simulink model "Constant_Load_NoStim_mt2"  (Simulink 6.6)
settings: Solver=FixedStepDiscrete  StartTime=0.0  StopTime=inf  FixedStep=parameters.model.sample_time  RelTol=1e-3
values from neighbouring files (symbols this model uses):
  animation =     [FESCycling_30_PRE_CONST_loaded_12Aug2014_085817.mat]
  cad_ref = 30    [FESCycling_30_PRE_CONST_loaded_12Aug2014_085817.mat]    (also in constant_load_load.m = str2double(get(bla,'String')); constant_load_load_Orig.m = str2double(get(bla,'String')); param.m; param_orig.m = 0)
  freq_range = 1022.16    [FESCycling_30_PRE_CONST_loaded_12Aug2014_085817.mat]    (also in constant_load_load.m; constant_load_load_Orig.m = 466.8; param.m; param_orig.m = 865.41)
  freq_zero = -38.15    [FESCycling_30_PRE_CONST_loaded_12Aug2014_085817.mat]    (also in constant_load_load.m; constant_load_load_Orig.m = 116.7756; param.m; param_orig.m = 39.49)
  parameters =     [FESCycling_30_PRE_CONST_loaded_12Aug2014_085817.mat]
  phio_mat = [1 -0.559 0.0775]    [FESCycling_30_PRE_CONST_loaded_12Aug2014_085817.mat]    (also in constant_load_load.m; constant_load_load_Orig.m; param.m; param_orig.m)
  Pstep = 5    [FESCycling_30_PRE_CONST_loaded_12Aug2014_085817.mat]    (also in constant_load_load.m = str2double(get(bla,'String')); constant_load_load_Orig.m = str2double(get(bla,'String')); param.m = 32; param_orig.m = 114)
  Pw = 0    [FESCycling_30_PRE_CONST_loaded_12Aug2014_085817.mat]    (also in constant_load_load.m = str2double(get(bla,'String')); constant_load_load_Orig.m = str2double(get(bla,'String')); param.m; param_orig.m)
  ro_mat = [0.7602 -0.2976 0.0591]    [FESCycling_30_PRE_CONST_loaded_12Aug2014_085817.mat]    (also in constant_load_load.m; constant_load_load_Orig.m; param.m; param_orig.m)
  s_mat = [0.0005025 -0.0003467]    [FESCycling_30_PRE_CONST_loaded_12Aug2014_085817.mat]    (also in constant_load_load.m = [0.5025 -0.3467]*1e-3; constant_load_load_Orig.m = [0.5025 -0.3467]*1e-3; param.m = [0.5025 -0.3467]*1e-3; param_orig.m = [0.5025 -0.3467]*1e-3)
  slope = 15.81    [FESCycling_30_PRE_CONST_loaded_12Aug2014_085817.mat]    (also in constant_load_load.m; constant_load_load_Orig.m = 14.1374; param.m; param_orig.m = 14.1374)
  stim_max = 0.1    [FESCycling_30_PRE_CONST_loaded_12Aug2014_085817.mat]    (also in constant_load_load.m; constant_load_load_Orig.m; param.m = 500; param_orig.m = 0)
  stim_min = 0    [FESCycling_30_PRE_CONST_loaded_12Aug2014_085817.mat]    (also in constant_load_load.m; constant_load_load_Orig.m; param.m; param_orig.m)
  t_mat = [0.0002987 -0.000166 2.31e-05]    [FESCycling_30_PRE_CONST_loaded_12Aug2014_085817.mat]    (also in constant_load_load.m = [0.2987 -0.1660 0.0231]*1e-3; constant_load_load_Orig.m = [0.2987 -0.1660 0.0231]*1e-3; param.m = [0.2987 -0.1660 0.0231]*1e-3; param_orig.m = [0.2987 -0.1660 0.0231]*1e-3)
  Ts = 20    [FESCycling_30_PRE_CONST_loaded_12Aug2014_085817.mat]    (also in constant_load_load.m; constant_load_load_Orig.m; param.m; param_orig.m)
  Tw = 6000    [FESCycling_30_PRE_CONST_loaded_12Aug2014_085817.mat]    (also in constant_load_load.m; constant_load_load_Orig.m; param.m; param_orig.m)
undefined symbols (not defined in the file or in its folder): ansim
libraries: ni_lib x2, Stimulation_Currents_lib x1, stimulation_staticAngles_lib x1
settings Model: Tag=D:\Ben\Matlab_Files\my_FES_Stuff\FES_Cycling_Models\Parameter_Files\GLA_BEN_Params_3.m  Creator=research  LastModifiedBy=research
settings DataIOCC: SignalLoggingName=sigsOut
settings OptimizationCC: BooleanDataType=off
settings DebuggingCC: SignalResolutionControl=TryResolveAllWithWarning  SolverPrmCheckMsg=none  MultiTaskDSMMsg=warning  MultiTaskCondExecSysMsg=none  StrictBusMsg=None
settings HardwareCC: TargetUnknown=on
settings RTWCC: IncludeERTFirstTime=on

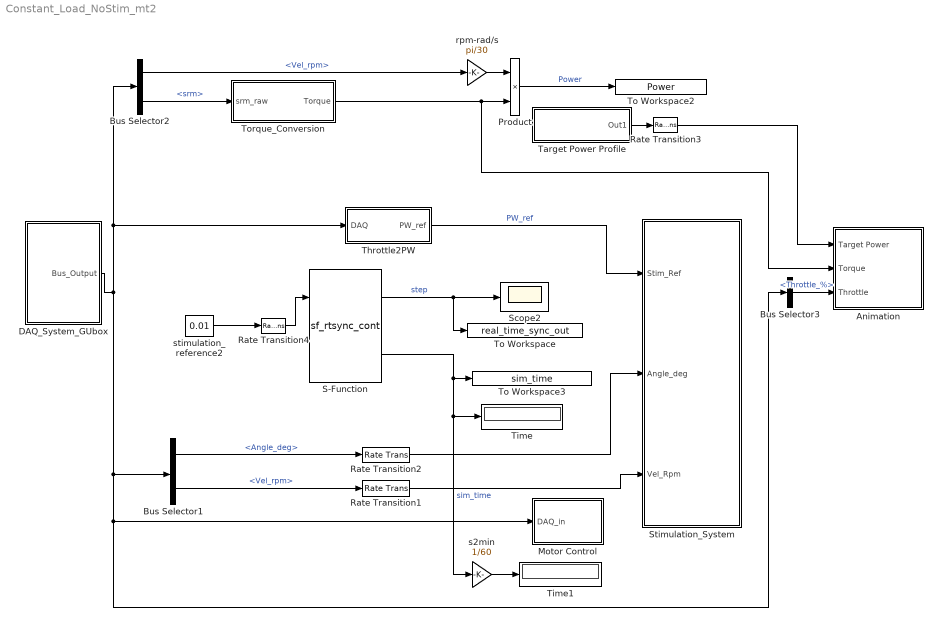
== system Constant_Load_NoStim_mt2 ==
  Animation : Subsystem
  Bus Selector1 : BusSelector  OutputSignals=Angle_deg,Vel_rpm
  Bus Selector2 : BusSelector  OutputSignals=Vel_rpm,srm
  Bus Selector3 : BusSelector  OutputSignals=Throttle_%
  DAQ_System_GUbox : Subsystem
  Motor Control : Subsystem
  Product : Product  SaturateOnIntegerOverflow=on
  Rate Transition1 : RateTransition  OutPortSampleTime=parameters.model.sample_time
  Rate Transition2 : RateTransition  OutPortSampleTime=parameters.model.sample_time
  Rate Transition3 : RateTransition  OutPortSampleTime=parameters.sample_time
  Rate Transition4 : RateTransition  X0=0.011  OutPortSampleTime=parameters.model.sample_time
  S-Function : S-Function  FunctionName=sf_rtsync_cont  Parameters=1
  Scope2 : Scope
      settings: YMin=-3.46945e-018  YMax=0.12
  Stimulation_System : Subsystem
  Target Power Profile : Subsystem
  Throttle2PW : Subsystem
  Time : Display
  Time1 : Display
  To Workspace : ToWorkspace  VariableName=real_time_sync_out  SampleTime=parameters.model.sample_time  SaveFormat=Array
  To Workspace2 : ToWorkspace  VariableName=Power  SampleTime=parameters.sample_time  SaveFormat=Array
  To Workspace3 : ToWorkspace  VariableName=sim_time  SampleTime=-1  SaveFormat=Array
      settings: Decimation=5
  Torque_Conversion : Subsystem
  rpm-rad/s : Gain  Gain=pi/30  SaturateOnIntegerOverflow=on
  s2min : Gain  Gain=1/60  SaturateOnIntegerOverflow=on
  stimulation_reference2 : Constant  Value=0.01
      mask Type: text(0.5,0.5,'bla_name.bla', 'VerticalAlignment', 'middle', 'HorizontalAlignment', 'centre')
  wires:
  Bus Selector1/2 -> Rate Transition1/1  "<Vel_rpm>"
  Bus Selector1/1 -> Rate Transition2/1  "<Angle_deg>"
  Bus Selector2/2 -> Torque_Conversion/1(srm_raw)  "<srm>"
  DAQ_System_GUbox/1(Bus_Output) -> Bus Selector1/1, Motor Control/1(DAQ_in), Bus Selector3/1, Bus Selector2/1, Throttle2PW/1(DAQ)
  Rate Transition1/1 -> Stimulation_System/3(Vel_Rpm)
  Rate Transition2/1 -> Stimulation_System/2(Angle_deg)
  S-Function/2 -> To Workspace3/1, Time/1, s2min/1  "sim_time"
  S-Function/1 -> Scope2/1, To Workspace/1  "step"
  Rate Transition4/1 -> S-Function/1
  stimulation_reference2/1 -> Rate Transition4/1
  s2min/1 -> Time1/1
  Torque_Conversion/1(Torque) -> Product/2, Animation/2(Torque)
  rpm-rad/s/1 -> Product/1
  Bus Selector2/1 -> rpm-rad/s/1  "<Vel_rpm>"
  Target Power Profile/1(Out1) -> Rate Transition3/1
  Product/1 -> To Workspace2/1  "Power"
  Rate Transition3/1 -> Animation/1(Target Power)
  Bus Selector3/1 -> Animation/3(Throttle)  "<Throttle_%>"
  Throttle2PW/1(PW_ref) -> Stimulation_System/1(Stim_Ref)  "PW_ref"

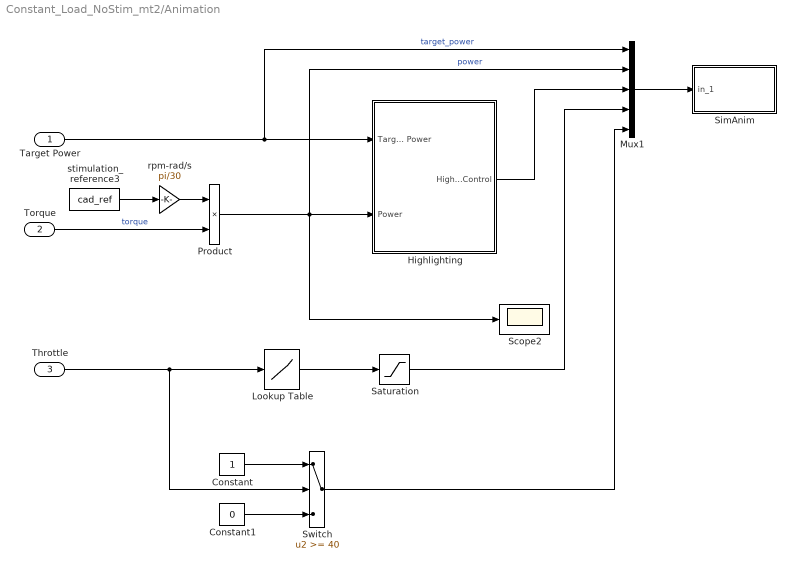
== system Constant_Load_NoStim_mt2/Animation ==
  Target Power : Inport
  Torque : Inport  Port=2
  Throttle : Inport  Port=3
  Constant : Constant
  Constant1 : Constant  Value=0
  Highlighting : Subsystem
  Lookup Table : Lookup  InputValues=[0 40 100]  OutputValues=[-5 0 19.9]
  Mux1 : Mux  Inputs=5
  Product : Product  SaturateOnIntegerOverflow=on
  Saturation : Saturate  UpperLimit=19.9  LowerLimit=-5
  Scope2 : Scope
      settings: TimeRange=2000  YMin=-2  YMax=60  SaveName=ScopeData6
  SimAnim : Subsystem
      settings: NameChangeFcn=ansim([],[],[],'NameChange');  OpenFcn=ansimini #Initialize
      mask Type: Simulation Animation
      mask Help: cal2.mat
      mask Display: disp('Simulation\nAnimation')
  Switch : Switch  Threshold=40
  rpm-rad/s : Gain  Gain=pi/30  SaturateOnIntegerOverflow=on
  stimulation_reference3 : Constant  Value=cad_ref
      mask Type: text(0.5,0.5,'bla_name.bla', 'VerticalAlignment', 'middle', 'HorizontalAlignment', 'centre')
  wires:
  Mux1/1 -> SimAnim/1(in_1)
  Target Power/1 -> Highlighting/1(Target Power), Mux1/1  "target_power"
  Highlighting/1(Highlight Control) -> Mux1/3
  Lookup Table/1 -> Saturation/1
  Saturation/1 -> Mux1/4
  Throttle/1 -> Lookup Table/1, Switch/2
  Constant/1 -> Switch/1
  Constant1/1 -> Switch/3
  Switch/1 -> Mux1/5
  rpm-rad/s/1 -> Product/1
  Product/1 -> Mux1/2, Highlighting/2(Power), Scope2/1  "power"
  Torque/1 -> Product/2  "torque"
  stimulation_reference3/1 -> rpm-rad/s/1

== system Constant_Load_NoStim_mt2/DAQ_System_GUbox ==
  note: Angle velocity (cadence) is more
      | useful in rpm (revolutions per
      | minute) so devide deg/s by 6.
  note: Convert the angle from between
      | 0 and 1 to between 0 and 360
      | and calculate the rate of change
      | of the angle in deg/s.
  Angle Conversion : Subsystem
  Bus Creator : BusCreator
  Bus Selector1 : BusSelector  OutputSignals=shaft_encoder_raw
  Bus Selector3 : BusSelector  OutputSignals=throttle_raw
  Gain1 : Gain  Gain=1/6  SaturateOnIntegerOverflow=on
  Hardware Interface via GU box : Subsystem
  Output Signal Conversion : Subsystem
  Output Signal Conversion2 : Subsystem
  Throttle Valuation : Subsystem
  To Workspace1 : ToWorkspace  VariableName=angle_deg  SampleTime=-1  SaveFormat=Array
  To Workspace2 : ToWorkspace  VariableName=vel_rpm  SampleTime=-1  SaveFormat=Array
  Bus_Output : Outport
  wires:
  Output Signal Conversion2/1(Out = 0 to 1) -> Throttle Valuation/1(throttle (0 to 1))
  Gain1/1 -> To Workspace2/1, Bus Creator/2  "Vel_rpm"
  Angle Conversion/2(Vel (deg/s)) -> Gain1/1
  Output Signal Conversion/1(Out = 0 to 1) -> Angle Conversion/1(Angle (0 to 1 volts))
  Bus Selector1/1 -> Output Signal Conversion/1(In = 0 to 5)  "<shaft_encoder_raw>"
  Bus Selector3/1 -> Output Signal Conversion2/1(In = 0 to 5)  "<throttle_raw>"
  Angle Conversion/1(Angle (deg)) -> To Workspace1/1, Bus Creator/1  "Angle_deg"
  Throttle Valuation/1(Throttle_%) -> Bus Creator/3  "Throttle_%"
  Hardware Interface via GU box/1(Hardware_Out_1) -> Bus Selector1/1, Bus Selector3/1
  Hardware Interface via GU box/2(Hardware_Out_3) -> Bus Creator/4  "srm"
  Bus Creator/1 -> Bus_Output/1

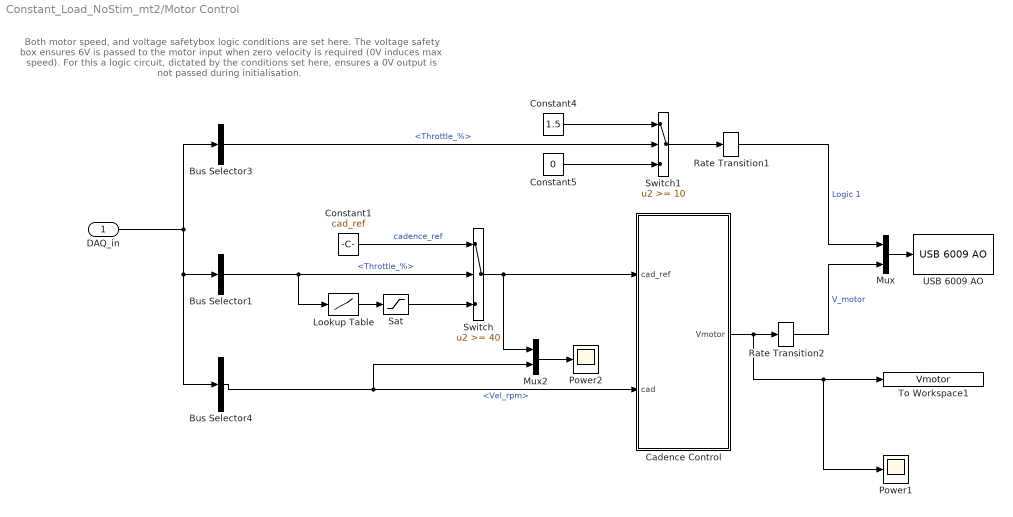
== system Constant_Load_NoStim_mt2/Motor Control ==
  note: Both motor speed, and voltage safetybox logic conditions are set here.
      | The voltage safety box ensures 6V is passed to the motor input when
      | zero velocity is required (0V induces max speed). For this a logic circuit,
      | dictated by the conditions set here, ensures a 0V output is not passed
      | during initialisation.
  DAQ_in : Inport
  Bus Selector1 : BusSelector  OutputSignals=Throttle_%
  Bus Selector3 : BusSelector  OutputSignals=Throttle_%
  Bus Selector4 : BusSelector  OutputSignals=Vel_rpm
  Cadence Control : Subsystem
  Constant1 : Constant  Value=cad_ref  SampleTime=-1
  Constant4 : Constant  Value=1.5
  Constant5 : Constant  Value=0
  Lookup Table : Lookup  InputValues=[10 40]  OutputValues=[0 cad_ref]  LookUpMeth=Interpolation-Use End Values
  Mux : Mux  Inputs=2
  Mux2 : Mux  Inputs=2
  Power1 : Scope
      settings: TimeRange=1000  YMin=0  SaveName=ScopeData3
  Power2 : Scope
      settings: TimeRange=1000  YMin=0  YMax=100  SaveName=ScopeData5
  Rate Transition1 : RateTransition  OutPortSampleTime=20
  Rate Transition2 : RateTransition  OutPortSampleTime=20
  Sat : Saturate  UpperLimit=cad_ref  LowerLimit=0
  Switch : Switch  Threshold=40
  Switch1 : Switch  Threshold=10
  To Workspace1 : ToWorkspace  VariableName=Vmotor  SampleTime=parameters.sample_time  SaveFormat=Array
  USB 6009 AO : ni_lib/USB 6009 AO  channels=[2 1]  Ts=20  inp_min=0  inp_max=5
  wires:
  DAQ_in/1 -> Bus Selector3/1, Bus Selector4/1, Bus Selector1/1
  Mux2/1 -> Power2/1
  Mux/1 -> USB 6009 AO/1
  Constant5/1 -> Switch1/3
  Switch1/1 -> Rate Transition1/1
  Constant4/1 -> Switch1/1
  Rate Transition1/1 -> Mux/1  "Logic 1"
  Rate Transition2/1 -> Mux/2  "V_motor"
  Bus Selector3/1 -> Switch1/2  "<Throttle_%>"
  Bus Selector4/1 -> Cadence Control/2(cad), Mux2/2  "<Vel_rpm>"
  Cadence Control/1(Vmotor) -> Rate Transition2/1, To Workspace1/1, Power1/1
  Switch/1 -> Cadence Control/1(cad_ref), Mux2/1
  Constant1/1 -> Switch/1  "cadence_ref"
  Bus Selector1/1 -> Switch/2, Lookup Table/1  "<Throttle_%>"
  Lookup Table/1 -> Sat/1
  Sat/1 -> Switch/3

== system Constant_Load_NoStim_mt2/Stimulation_System ==
  Stim_Ref : Inport
  Angle_deg : Inport  Port=2
  Vel_Rpm : Inport  Port=3
  Serial_Stimulation_System : Subsystem
  wires:
  Stim_Ref/1 -> Serial_Stimulation_System/1(Stim_ref)
  Angle_deg/1 -> Serial_Stimulation_System/2(Angle_deg)
  Vel_Rpm/1 -> Serial_Stimulation_System/3(Vel_rpm)

== system Constant_Load_NoStim_mt2/Target Power Profile ==
  Step : Step  Time=Tw  Before=Pw  After=Pw + Pstep  SampleTime=0
  Out1 : Outport
  wires:
  Step/1 -> Out1/1

== system Constant_Load_NoStim_mt2/Throttle2PW ==
  DAQ : Inport
  Bus Selector3 : BusSelector  OutputSignals=Throttle_%
  Lookup Table2 : Lookup  InputValues=[0 20 40 100]  OutputValues=[0 0 stim_min stim_max]  LookUpMeth=Interpolation-Use End Values
  Mux1 : Mux  Inputs=2
  Rate Transition1 : RateTransition  OutPortSampleTime=parameters.model.sample_time
  Saturation : Saturate  UpperLimit=stim_max  LowerLimit=0
  PW_ref : Outport
  wires:
  DAQ/1 -> Bus Selector3/1
  Bus Selector3/1 -> Rate Transition1/1  "<Throttle_%>"
  Mux1/1 -> PW_ref/1
  Rate Transition1/1 -> Lookup Table2/1
  Lookup Table2/1 -> Saturation/1
  Saturation/1 -> Mux1/1, Mux1/2  "pw_h_g"

== system Constant_Load_NoStim_mt2/Torque_Conversion ==
  srm_raw : Inport
  Discrete Transfer Fcn : DiscreteTransferFcn  Numerator="[0.0051    0.0101    0.0051]"  Denominator="[1.0000   -1.7889    0.8092]"  SampleTime=parameters.sample_time
  Mux : Mux  Inputs=2
  Normalise srm raw : Gain  Gain=1/5  SaturateOnIntegerOverflow=on
  SRM frequency - Voltage1 : Subsystem
  To Workspace2 : ToWorkspace  VariableName=Torque  SampleTime=parameters.sample_time  SaveFormat=Array
  torque : Scope
      settings: YMin=8.95  YMax=9.6  SaveName=ScopeData4
  Torque : Outport
  wires:
  srm_raw/1 -> Normalise srm raw/1
  SRM frequency - Voltage1/1(Torque (Nm)) -> Mux/1, Discrete Transfer Fcn/1  "torque_raw"
  Mux/1 -> torque/1
  Discrete Transfer Fcn/1 -> Mux/2, To Workspace2/1, Torque/1  "torque_(filtered)"
  Normalise srm raw/1 -> SRM frequency - Voltage1/1(In 0 to 1)

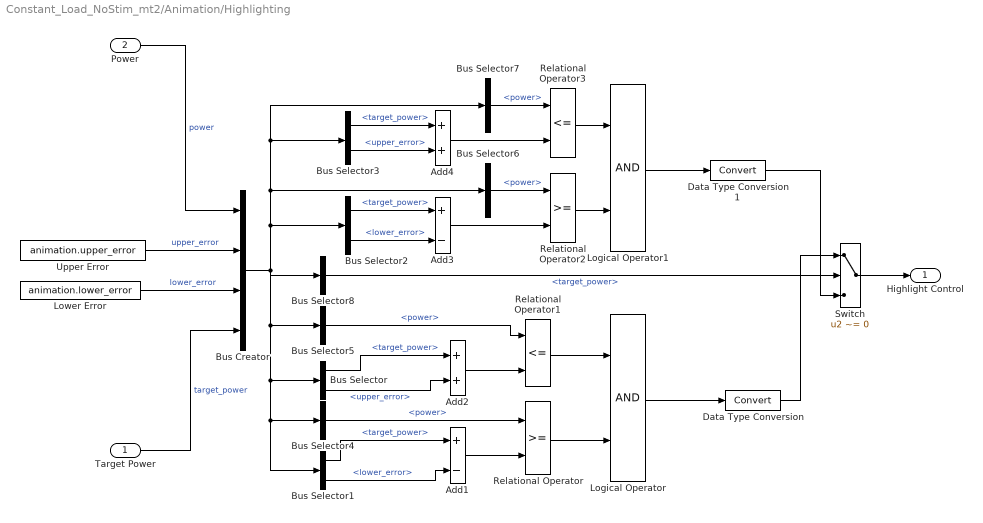
== system Constant_Load_NoStim_mt2/Animation/Highlighting ==
  Target Power : Inport
  Power : Inport  Port=2
  Add1 : Sum  Inputs=+-  OutScaling=2^-10
  Add2 : Sum  OutScaling=2^-10
  Add3 : Sum  Inputs=+-  OutScaling=2^-10
  Add4 : Sum  OutScaling=2^-10
  Bus Creator : BusCreator
  Bus Selector : BusSelector  OutputSignals=target_power,upper_error
  Bus Selector1 : BusSelector  OutputSignals=target_power,lower_error
  Bus Selector2 : BusSelector  OutputSignals=target_power,lower_error
  Bus Selector3 : BusSelector  OutputSignals=target_power,upper_error
  Bus Selector{4..7} (4 alike) : BusSelector  OutputSignals=power
  Bus Selector8 : BusSelector  OutputSignals=target_power
  Data Type Conversion : DataTypeConversion  OutDataTypeMode=double
  Data Type Conversion1 : DataTypeConversion  OutDataTypeMode=double
  Logical Operator : Logic  AllPortsSameDT=off  OutDataTypeMode=Boolean
  Logical Operator1 : Logic  AllPortsSameDT=off  OutDataTypeMode=Boolean
  Lower Error : Constant  Value=animation.lower_error
  Relational Operator : RelationalOperator  LogicOutDataTypeMode=Boolean
  Relational Operator1 : RelationalOperator  Operator=<=  LogicOutDataTypeMode=Boolean
  Relational Operator2 : RelationalOperator  LogicOutDataTypeMode=Boolean
  Relational Operator3 : RelationalOperator  Operator=<=  LogicOutDataTypeMode=Boolean
  Switch : Switch  Criteria=u2 ~= 0
  Upper Error : Constant  Value=animation.upper_error
  Highlight Control : Outport
  wires:
  Relational Operator/1 -> Logical Operator/2
  Logical Operator/1 -> Data Type Conversion/1
  Data Type Conversion/1 -> Switch/1
  Add1/1 -> Relational Operator/2
  Relational Operator3/1 -> Logical Operator1/1
  Relational Operator2/1 -> Logical Operator1/2
  Add4/1 -> Relational Operator3/2
  Add3/1 -> Relational Operator2/2
  Target Power/1 -> Bus Creator/4  "target_power"
  Bus Selector/1 -> Add2/1  "<target_power>"
  Bus Selector/2 -> Add2/2  "<upper_error>"
  Bus Creator/1 -> Bus Selector2/1, Bus Selector6/1, Bus Selector3/1, Bus Selector7/1, Bus Selector/1, Bus Selector4/1, Bus Selector1/1, Bus Selector5/1, Bus Selector8/1
  Bus Selector1/1 -> Add1/1  "<target_power>"
  Bus Selector1/2 -> Add1/2  "<lower_error>"
  Bus Selector2/1 -> Add3/1  "<target_power>"
  Bus Selector2/2 -> Add3/2  "<lower_error>"
  Bus Selector3/1 -> Add4/1  "<target_power>"
  Bus Selector3/2 -> Add4/2  "<upper_error>"
  Lower Error/1 -> Bus Creator/3  "lower_error"
  Upper Error/1 -> Bus Creator/2  "upper_error"
  Bus Selector7/1 -> Relational Operator3/1  "<power>"
  Bus Selector6/1 -> Relational Operator2/1  "<power>"
  Bus Selector5/1 -> Relational Operator1/1  "<power>"
  Bus Selector4/1 -> Relational Operator/1  "<power>"
  Logical Operator1/1 -> Data Type Conversion1/1
  Bus Selector8/1 -> Switch/2  "<target_power>"
  Data Type Conversion1/1 -> Switch/3
  Switch/1 -> Highlight Control/1
  Add2/1 -> Relational Operator1/2
  Relational Operator1/1 -> Logical Operator/1
  Power/1 -> Bus Creator/1  "power"

== system Constant_Load_NoStim_mt2/Animation/SimAnim ==
  in_1 : Inport
  Terminator : Terminator
  ansim : S-Function  LoadFcn=ansim([],[],[],'LoadBlock');  StartFcn=ansim([],[],[],'Start');  StopFcn=ansim([],[],[],'Stop');  FunctionName=ansim  Parameters=1
      settings: CopyFcn=ansim([],[],[],'CopyBlock');  DeleteFcn=ansim([],[],[],'DeleteBlock');
  wires:
  in_1/1 -> ansim/1
  ansim/1 -> Terminator/1

== system Constant_Load_NoStim_mt2/DAQ_System_GUbox/Angle Conversion ==
  note: This system converts an
      | angle described as a voltage
      | between 0 and 1 and turns it
      | into an angle in degrees.
      | The rate of change of angle
      | is also calculated.
  note: Ensure that the final angle
      | value is between 0 and 360
  note: Use this constant input
      | when the 0 point of the
      | input angle is not the same
      | as the 0 point needed by
      | the rest of the simulaink
      | model.
      | (left leg horizontally forward)
  note: Angle Conversion
  Angle (0 to 1 volts) : Inport
  0 < u < 360 : Fcn  Expr=u - 360*floor(u/360)
  Angle Derivative : Subsystem  mask(AngleDer){Tdf=0.5, Ts=5}
      mask prompts: Tdf "Filter constant"; Ts "Sampling Time"
      mask help:
      | This block calculates the angular velocity from the angle measuremet.  If the input angle is in degrees then the output velocity is in deg/s.  The block takes account of the transition from 359 deg to 0 deg or vice versa and computes the derivative based on the sample time given  The output is passed through a low pass filter based on the fliter constant also given.
      |
      | Implemented by Nils-Otto Negaard
      | Documented by Ben Saunders (17/06/2003)
  Angle Shift : Constant  Value=parameters.angle_shift
  Sum : Sum  Inputs=++|  SaturateOnIntegerOverflow=on  InputSameDT=on
  angle into degrees : Fcn  Expr=u*360
  Angle (deg) : Outport
  Vel (deg/s) : Outport  Port=2
  wires:
  angle into degrees/1 -> Angle Derivative/1(Angle), Sum/2
  Sum/1 -> 0 < u < 360/1
  0 < u < 360/1 -> Angle (deg)/1
  Angle (0 to 1 volts)/1 -> angle into degrees/1
  Angle Derivative/1(Vel (deg/s)) -> Vel (deg/s)/1
  Angle Shift/1 -> Sum/1

== system Constant_Load_NoStim_mt2/DAQ_System_GUbox/Hardware Interface via GU box ==
  note: Hardware Interface (via USB-6009)
  Bus Creator : BusCreator
  Demux1 : Demux  Outputs=5
  To Workspace1 : ToWorkspace  VariableName=throttle_raw  SampleTime=-1  SaveFormat=Array
  To Workspace2 : ToWorkspace  VariableName=srm_cad  SampleTime=-1  SaveFormat=Array
  To Workspace3 : ToWorkspace  VariableName=torque_dig  SampleTime=-1  SaveFormat=Array
  To Workspace4 : ToWorkspace  VariableName=torque_ana  SampleTime=-1  SaveFormat=Array
  To Workspace5 : ToWorkspace  VariableName=shaft_encoder_raw  SampleTime=-1  SaveFormat=Array
  USB 6009 AI : ni_lib/USB 6009 AI  channels=[1 2 3 4 5]  Ts=5  inp_min=-5  inp_max=5  terminalcfg=RSE
  Hardware_Out_1 : Outport
  Hardware_Out_3 : Outport  Port=2
  wires:
  Bus Creator/1 -> Hardware_Out_1/1
  Demux1/2 -> Bus Creator/2, To Workspace1/1  "throttle_raw"
  Demux1/5 -> To Workspace2/1  "srm_cadence"
  USB 6009 AI/1 -> Demux1/1
  Demux1/4 -> Bus Creator/4, To Workspace3/1  "torque_dig"
  Demux1/3 -> To Workspace4/1, Hardware_Out_3/1, Bus Creator/3  "torque_ana"
  Demux1/1 -> Bus Creator/1, To Workspace5/1  "shaft_encoder_raw"

== system Constant_Load_NoStim_mt2/DAQ_System_GUbox/Output Signal Conversion ==
  In = 0 to 5 : Inport
  Constant : Constant  Value=0
  Gain4 : Gain  Gain=1/5  SaturateOnIntegerOverflow=on
  Sum : Sum  Inputs=++|  SaturateOnIntegerOverflow=on  InputSameDT=on
  Out = 0 to 1 : Outport
  wires:
  In = 0 to 5/1 -> Gain4/1
  Sum/1 -> Out = 0 to 1/1
  Constant/1 -> Sum/1
  Gain4/1 -> Sum/2

== system Constant_Load_NoStim_mt2/DAQ_System_GUbox/Output Signal Conversion2 ==
  In = 0 to 5 : Inport
  Constant : Constant  Value=0
  Gain4 : Gain  Gain=1/5  SaturateOnIntegerOverflow=on
  Sum : Sum  Inputs=++|  SaturateOnIntegerOverflow=on  InputSameDT=on
  Out = 0 to 1 : Outport
  wires:
  In = 0 to 5/1 -> Gain4/1
  Sum/1 -> Out = 0 to 1/1
  Constant/1 -> Sum/1
  Gain4/1 -> Sum/2

== system Constant_Load_NoStim_mt2/DAQ_System_GUbox/Throttle Valuation ==
  note: Throttle Valuation
  note: This Subsystem is used to
      | scale the throttle signal from
      | an input of 0 to 1 to a
      | percentage (0 to 100).  Since
      | the throttle does not always
      | show 0 when let go, it is
      | forced to 0 using the validity
      | signal. This is a safty
      | consideration.  Note that
      | when the throttle switch is on
      | then the validity signal still
      | goes to 0 when the throttle
      | has been let go.
  throttle (0 to 1) : Inport
  Gain3 : Gain  Gain=100  SaturateOnIntegerOverflow=on
  Throttle_% : Outport
  wires:
  Gain3/1 -> Throttle_%/1  "Throttle_%"
  throttle (0 to 1)/1 -> Gain3/1

== system Constant_Load_NoStim_mt2/Motor Control/Cadence Control ==
  cad_ref : Inport
  cad : Inport  Port=2
  Gain1 : Gain  Gain=6  SaturateOnIntegerOverflow=on
  Gain2 : Gain  Gain=6  SaturateOnIntegerOverflow=on
  Lookup Table : Lookup  InputValues=[0 1]  OutputValues=[2.5 1.25]
  Rate Transition1 : RateTransition  OutPortSampleTime=parameters.sample_time
  rstcon antireset2 : Subsystem
  Vmotor : Outport
  wires:
  rstcon antireset2/1(Vm_ref) -> Lookup Table/1
  cad/1 -> Gain1/1
  Gain2/1 -> rstcon antireset2/1(cad_ref)
  cad_ref/1 -> Gain2/1
  Lookup Table/1 -> Rate Transition1/1
  Gain1/1 -> rstcon antireset2/2(cad_act)
  Rate Transition1/1 -> Vmotor/1

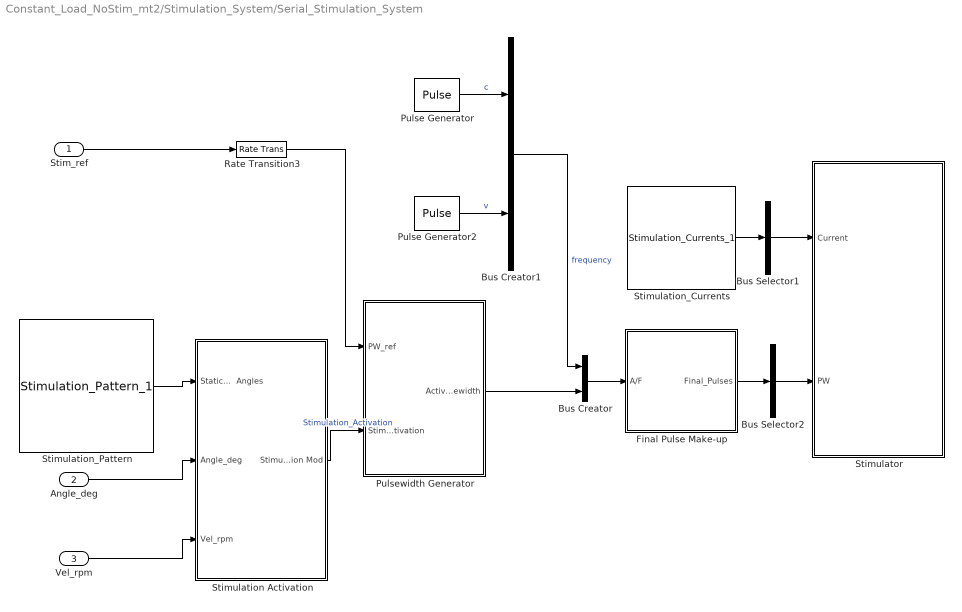
== system Constant_Load_NoStim_mt2/Stimulation_System/Serial_Stimulation_System ==
  Stim_ref : Inport
  Angle_deg : Inport  Port=2
  Vel_rpm : Inport  Port=3
  Bus Creator : BusCreator  Inputs=2
  Bus Creator1 : BusCreator  Inputs=2
  Bus Selector1 : BusSelector  OutputSignals=R.Quad,R.Ham,R.Glut,L.Quad,L.Ham,L.Glut  OutputAsBus=on
  Bus Selector2 : BusSelector  OutputSignals=R.Quad_r,R.Ham_r,R.Glut_r,L.Quad_l,L.Ham_l,L.Glut_l  OutputAsBus=on
  Final Pulse Make-up : Subsystem
  Pulse Generator : DiscretePulseGenerator  Period=3
  Pulse Generator2 : DiscretePulseGenerator  Period=3
  Pulsewidth Generator : Subsystem
  Rate Transition3 : RateTransition  OutPortSampleTime=parameters.model.sample_time
  Stimulation Activation : Subsystem
  Stimulation_Currents : Stimulation_Currents_lib/Stimulation_Currents_1  SystemSampleTime=-1  Quad_R=40  Ham_R=0  Glut_R=0  Calf_R=0  ExactOpp=on  Quad_L=[40]  Ham_L=[0]  Glut_L=[0]  Calf_L=[0]
  Stimulation_Pattern : stimulation_staticAngles_lib/Stimulation_Pattern_1  SystemSampleTime=-1  Quad_R=[55 155]  Ham_R=[188 265]  Glut_R=[90 180]  Calf_R=[180 205]  ExactOpp=on  Quad_L="[235  335]"  Ham_L="[8  85]"  Glut_L="[270    0]"  Calf_L="[0  25]"
  Stimulator : Subsystem
  wires:
  Stimulation Activation/1(Stimulation  Activation Mod) -> Pulsewidth Generator/2(Stimulation Activation)  "Stimulation_Activation"
  Stimulation_Pattern/1 -> Stimulation Activation/1(Static  Stimulation  Angles)
  Angle_deg/1 -> Stimulation Activation/2(Angle_deg)
  Vel_rpm/1 -> Stimulation Activation/3(Vel_rpm)
  Stimulation_Currents/1 -> Bus Selector1/1
  Stim_ref/1 -> Rate Transition3/1
  Rate Transition3/1 -> Pulsewidth Generator/1(PW_ref)
  Bus Selector1/1 -> Stimulator/1(Current)
  Bus Selector2/1 -> Stimulator/2(PW)
  Pulse Generator2/1 -> Bus Creator1/2  "v"
  Pulse Generator/1 -> Bus Creator1/1  "c"
  Bus Creator1/1 -> Bus Creator/1  "frequency"
  Final Pulse Make-up/1(Final_Pulses) -> Bus Selector2/1
  Bus Creator/1 -> Final Pulse Make-up/1(A/F)
  Pulsewidth Generator/1(Activation/Pulsewidth) -> Bus Creator/2

== system Constant_Load_NoStim_mt2/Torque_Conversion/SRM frequency - Voltage1 ==
  note: Convert frequency to Torque (Nm)
      |
      | The data for this can be gained
      | from the SRM sensot itself. The
      | ZOPM (Zero Offset of the Power
      | Meter) is calculated and displayed
      | by the SRM meter.  Please check
      | the SRM manual for details. The
      | 'Slope' value can be read from the
      | back of the SRM sensor.
  note: SRM Frequency to Voltage
  note: This system reads in a 0 to 1 voltage
      | from an AD card that comes from a
      | frequency to voltage converter.  The
      | frequency signal comes from the SRM
      | sensor meter.  In order to work out the
      | torque on the sensor the process has
      | to be reversed.  Thus the voltage has
      | to be converted back into a frequency
      | and then back into a torque.
  note: Convert signal to frequency
      |
      | The frequency to voltage converter
      | was designed (at Glasgow by
      | Gordon) such that 0 volts = 300 Hz
      | and 5 volts = 1000 Hz.  The
      | mapping is linear.
  note: The final signal is filtered.
      | This may have a relatively
      | large rise time so that
      | cyclinc pedal forces are
      | smoothrd out. (ie forces at
      | 90 deg will always be
      | different to forces at 180
      | deg).
  In 0 to 1 : Inport
  1 / Slope1 : Constant  Value=1/slope
  Frequency Range : Constant  Value=freq_range
  Product : Product  SaturateOnIntegerOverflow=on  InputSameDT=on
  Product1 : Product  SaturateOnIntegerOverflow=on  InputSameDT=on
  Sum : Sum  Inputs=|++  SaturateOnIntegerOverflow=on  InputSameDT=on
  Sum1 : Sum  Inputs=-+|  SaturateOnIntegerOverflow=on  InputSameDT=on
  Sum2 : Sum  Inputs=-+|  SaturateOnIntegerOverflow=on  InputSameDT=on
  ZOPM : Constant  Value=parameters.srm_conversion.ZOPM
  Zero Frequency : Constant  Value=freq_zero
  offset : Constant  Value=-9
  Torque (Nm) : Outport
  wires:
  Zero Frequency/1 -> Sum/2
  1 / Slope1/1 -> Product1/2
  ZOPM/1 -> Sum2/1
  Frequency Range/1 -> Product/1
  Sum/1 -> Sum2/2  "frequency"
  In 0 to 1/1 -> Product/2
  Product/1 -> Sum/1
  Sum2/1 -> Product1/1
  Product1/1 -> Sum1/2  "Nm"
  Sum1/1 -> Torque (Nm)/1
  offset/1 -> Sum1/1

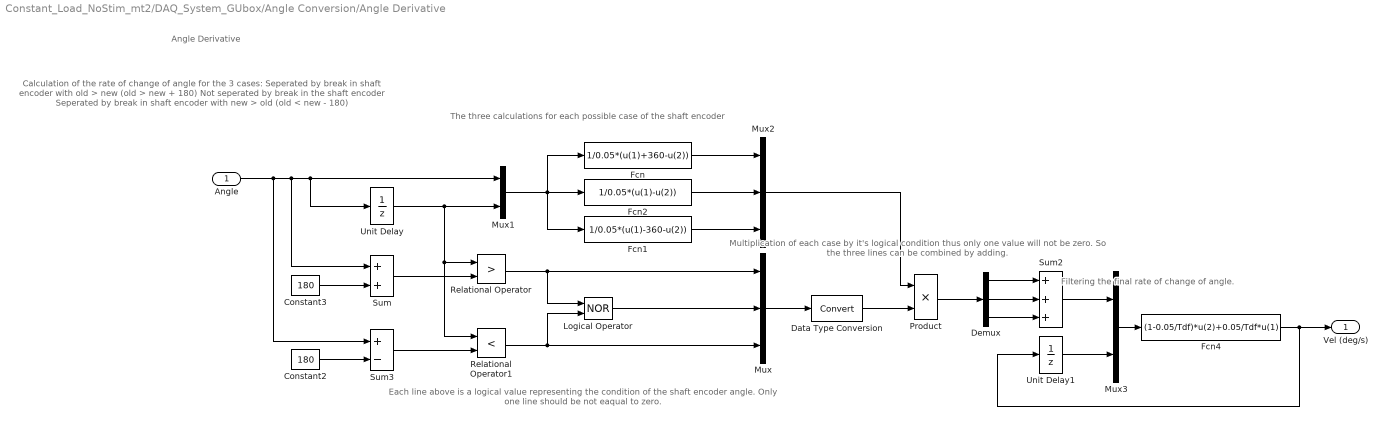
== system Constant_Load_NoStim_mt2/DAQ_System_GUbox/Angle Conversion/Angle Derivative ==
  note: Calculation of the rate of change of angle
      | for the 3 cases:
      | Seperated by break in shaft encoder with old > new (old > new + 180)
      | Not seperated by break in the shaft encoder
      | Seperated by break in shaft encoder with new > old (old < new - 180)
  note: Each line above is a logical value
      | representing the condition of the
      | shaft encoder angle.  Only one line
      | should be not eaqual to zero.
  note: The three calculations for each
      | possible case of the shaft encoder
  note: Multiplication of each case
      | by it's logical condition thus
      | only one value will not be zero.
      | So the three lines can be
      | combined by adding.
  note: Filtering the final rate of
      | change of angle.
  note: Angle Derivative
  Angle : Inport
  Constant2 : Constant  Value=180  VectorParams1D=off
  Constant3 : Constant  Value=180  VectorParams1D=off
  Data Type Conversion : DataTypeConversion  OutDataTypeMode=double  SaturateOnIntegerOverflow=on  RndMeth=Zero
  Demux : Demux  Outputs=3
  Fcn : Fcn  Expr=1/0.05*(u(1)+360-u(2))
  Fcn1 : Fcn  Expr=1/0.05*(u(1)-360-u(2))
  Fcn2 : Fcn  Expr=1/0.05*(u(1)-u(2))
  Fcn4 : Fcn  Expr=(1-0.05/Tdf)*u(2)+0.05/Tdf*u(1)
  Logical Operator : Logic  Operator=NOR
  Mux : Mux  Inputs=3
  Mux1 : Mux  Inputs=2
  Mux2 : Mux  Inputs=3
  Mux3 : Mux  Inputs=2
  Product : Product  SaturateOnIntegerOverflow=on  InputSameDT=on
  Relational Operator : RelationalOperator  Operator=>  InputSameDT=on
  Relational Operator1 : RelationalOperator  Operator=<  InputSameDT=on
  Sum : Sum  SaturateOnIntegerOverflow=on  InputSameDT=on
  Sum2 : Sum  Inputs=+++  SaturateOnIntegerOverflow=on  InputSameDT=on
  Sum3 : Sum  Inputs=+-  SaturateOnIntegerOverflow=on  InputSameDT=on
  Unit Delay : UnitDelay  SampleTime=-1
  Unit Delay1 : UnitDelay  SampleTime=Ts
  Vel (deg/s) : Outport
  wires:
  Data Type Conversion/1 -> Product/2
  Unit Delay/1 -> Mux1/2, Relational Operator1/1, Relational Operator/1
  Sum/1 -> Relational Operator/2
  Constant2/1 -> Sum3/2
  Relational Operator1/1 -> Logical Operator/2, Mux/3
  Relational Operator/1 -> Logical Operator/1, Mux/1
  Mux/1 -> Data Type Conversion/1
  Mux1/1 -> Fcn/1, Fcn1/1, Fcn2/1
  Fcn/1 -> Mux2/1
  Mux2/1 -> Product/1
  Fcn4/1 -> Vel (deg/s)/1, Unit Delay1/1
  Mux3/1 -> Fcn4/1
  Unit Delay1/1 -> Mux3/2
  Product/1 -> Demux/1
  Demux/1 -> Sum2/1
  Demux/2 -> Sum2/2
  Demux/3 -> Sum2/3
  Sum2/1 -> Mux3/1
  Angle/1 -> Sum3/1, Sum/1, Unit Delay/1, Mux1/1
  Constant3/1 -> Sum/2
  Sum3/1 -> Relational Operator1/2
  Logical Operator/1 -> Mux/2
  Fcn2/1 -> Mux2/2
  Fcn1/1 -> Mux2/3

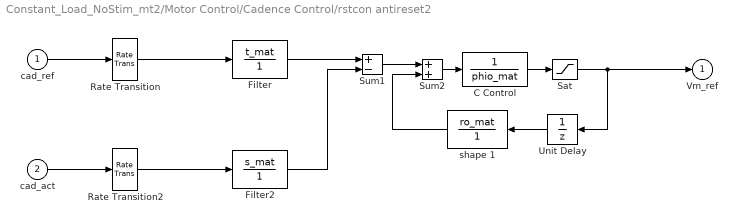
== system Constant_Load_NoStim_mt2/Motor Control/Cadence Control/rstcon antireset2 ==
  cad_ref : Inport
  cad_act : Inport  Port=2
  C Control : DiscreteFilter  Numerator=1  Denominator=phio_mat  SampleTime=Ts
  Filter : DiscreteFilter  Numerator=t_mat  Denominator=1  SampleTime=Ts
  Filter2 : DiscreteFilter  Numerator=s_mat  Denominator=1  SampleTime=Ts
  Rate Transition : RateTransition  OutPortSampleTime=Ts
  Rate Transition2 : RateTransition  OutPortSampleTime=Ts
  Sat : Saturate  UpperLimit=1  LowerLimit=0
  Sum1 : Sum  Inputs=+-  SaturateOnIntegerOverflow=on  InputSameDT=on
  Sum2 : Sum  SaturateOnIntegerOverflow=on  InputSameDT=on
  Unit Delay : UnitDelay  Orientation=left  SampleTime=Ts
  shape 1 : DiscreteFilter  Orientation=left  Numerator=ro_mat  Denominator=1  SampleTime=Ts
  Vm_ref : Outport  InitialOutput=0
  wires:
  cad_ref/1 -> Rate Transition/1
  Unit Delay/1 -> shape 1/1
  Sat/1 -> Unit Delay/1, Vm_ref/1
  Sum2/1 -> C Control/1
  C Control/1 -> Sat/1
  shape 1/1 -> Sum2/2
  Filter/1 -> Sum1/1
  Sum1/1 -> Sum2/1
  Rate Transition/1 -> Filter/1
  cad_act/1 -> Rate Transition2/1
  Rate Transition2/1 -> Filter2/1
  Filter2/1 -> Sum1/2

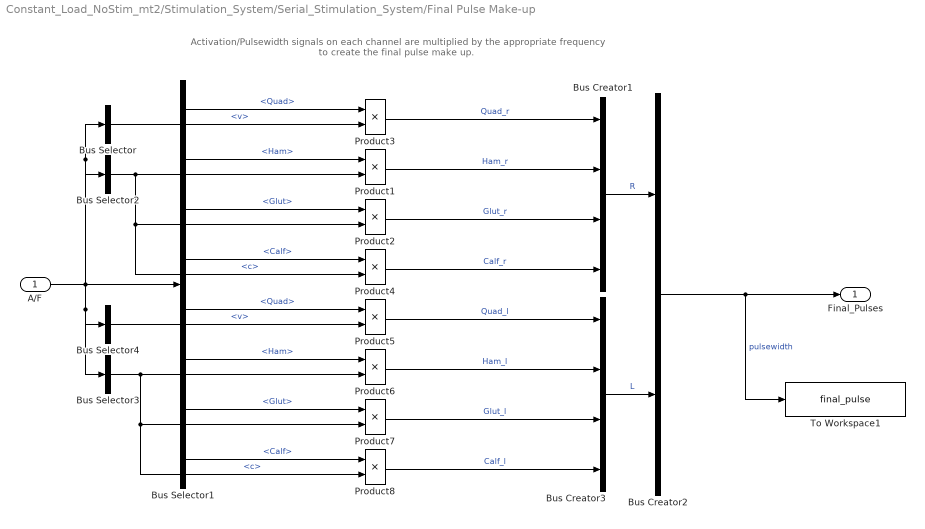
== system Constant_Load_NoStim_mt2/Stimulation_System/Serial_Stimulation_System/Final Pulse Make-up ==
  note: Activation/Pulsewidth signals on each channel are multiplied
      | by the appropriate frequency to create the final pulse make up.
  A/F : Inport
  Bus Creator1 : BusCreator
  Bus Creator2 : BusCreator  Inputs=2
  Bus Creator3 : BusCreator
  Bus Selector : BusSelector  OutputSignals=frequency.v
  Bus Selector1 : BusSelector  OutputSignals=pulsewidth.R.Quad,pulsewidth.R.Ham,pulsewidth.R.Glut,pulsewidth.R.Calf,pulsewidth.L.Quad,pulsewidth.L.Ham,pulsewidth.L.Glut,pulsewidth.L.Calf
  Bus Selector2 : BusSelector  OutputSignals=frequency.c
  Bus Selector3 : BusSelector  OutputSignals=frequency.c
  Bus Selector4 : BusSelector  OutputSignals=frequency.v
  Product{1..8} (8 alike) : Product  SaturateOnIntegerOverflow=on  InputSameDT=on
  To Workspace1 : ToWorkspace  VariableName=final_pulse  SampleTime=parameters.model.sample_time  SaveFormat=Array
      settings: Decimation=5
  Final_Pulses : Outport
  wires:
  Bus Creator2/1 -> Final_Pulses/1, To Workspace1/1  "pulsewidth"
  Bus Creator3/1 -> Bus Creator2/2  "L"
  Bus Creator1/1 -> Bus Creator2/1  "R"
  A/F/1 -> Bus Selector1/1, Bus Selector/1, Bus Selector2/1, Bus Selector3/1, Bus Selector4/1
  Bus Selector1/1 -> Product3/1  "<Quad>"
  Bus Selector/1 -> Product3/2  "<v>"
  Bus Selector1/2 -> Product1/1  "<Ham>"
  Bus Selector2/1 -> Product1/2, Product2/2, Product4/2  "<c>"
  Bus Selector1/3 -> Product2/1  "<Glut>"
  Bus Selector1/4 -> Product4/1  "<Calf>"
  Bus Selector1/5 -> Product5/1  "<Quad>"
  Bus Selector1/6 -> Product6/1  "<Ham>"
  Bus Selector1/7 -> Product7/1  "<Glut>"
  Bus Selector1/8 -> Product8/1  "<Calf>"
  Bus Selector4/1 -> Product5/2  "<v>"
  Bus Selector3/1 -> Product6/2, Product7/2, Product8/2  "<c>"
  Product3/1 -> Bus Creator1/1  "Quad_r"
  Product1/1 -> Bus Creator1/2  "Ham_r"
  Product2/1 -> Bus Creator1/3  "Glut_r"
  Product4/1 -> Bus Creator1/4  "Calf_r"
  Product5/1 -> Bus Creator3/1  "Quad_l"
  Product6/1 -> Bus Creator3/2  "Ham_l"
  Product7/1 -> Bus Creator3/3  "Glut_l"
  Product8/1 -> Bus Creator3/4  "Calf_l"

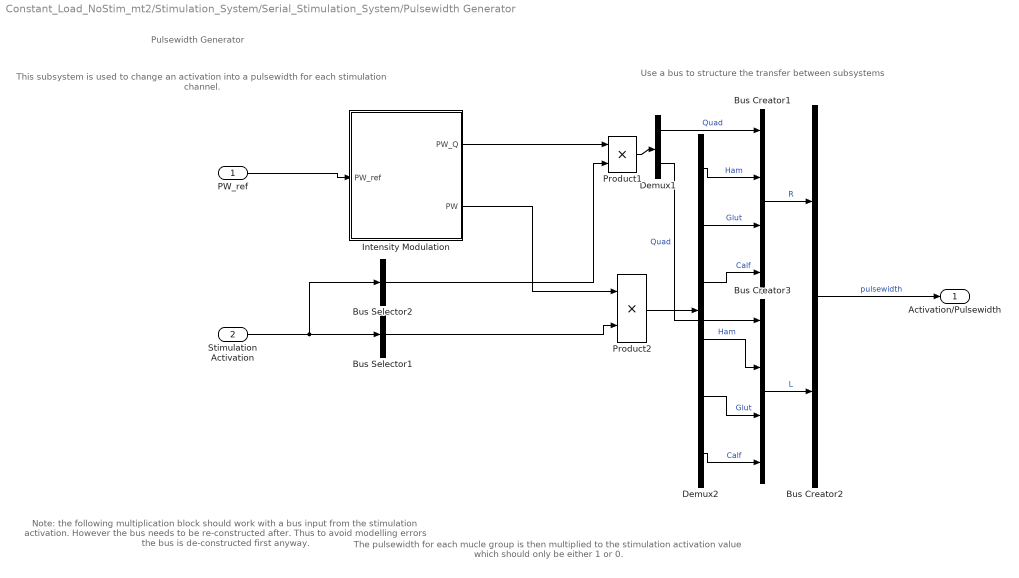
== system Constant_Load_NoStim_mt2/Stimulation_System/Serial_Stimulation_System/Pulsewidth Generator ==
  note: Pulsewidth Generator
  note: This subsystem is used to change
      | an activation into a pulsewidth for
      | each stimulation channel.
  note: Note: the following multiplication
      | block should work with a bus input
      | from the stimulation activation.
      | However the bus needs to be
      | re-constructed after.  Thus to
      | avoid modelling errors the bus is
      | de-constructed first anyway.
  note: The pulsewidth for each
      | mucle group is then
      | multiplied to the stimulation
      | activation value which
      | should only be either 1 or 0.
  note: Use a bus to structure the
      | transfer between subsystems
  PW_ref : Inport
  Stimulation Activation : Inport  Port=2
  Bus Creator1 : BusCreator
  Bus Creator2 : BusCreator  Inputs=2
  Bus Creator3 : BusCreator
  Bus Selector1 : BusSelector  OutputSignals=R.Ham,R.Glut,R.Calf,L.Ham,L.Glut,L.Calf  OutputAsBus=on
  Bus Selector2 : BusSelector  OutputSignals=R.Quad,L.Quad  OutputAsBus=on
  Demux1 : Demux  Outputs=2
  Demux2 : Demux  Outputs=6
  Intensity Modulation : Subsystem
  Product1 : Product  SaturateOnIntegerOverflow=on  InputSameDT=on
  Product2 : Product  SaturateOnIntegerOverflow=on  InputSameDT=on
  Activation/Pulsewidth : Outport
  wires:
  Stimulation Activation/1 -> Bus Selector1/1, Bus Selector2/1
  Bus Creator1/1 -> Bus Creator2/1  "R"
  Bus Creator3/1 -> Bus Creator2/2  "L"
  Bus Creator2/1 -> Activation/Pulsewidth/1  "pulsewidth"
  Bus Selector1/1 -> Product2/2
  Product2/1 -> Demux2/1
  PW_ref/1 -> Intensity Modulation/1(PW_ref)
  Intensity Modulation/2(PW) -> Product2/1
  Demux2/6 -> Bus Creator3/4  "Calf"
  Demux2/5 -> Bus Creator3/3  "Glut"
  Demux2/4 -> Bus Creator3/2  "Ham"
  Bus Selector2/1 -> Product1/2
  Intensity Modulation/1(PW_Q) -> Product1/1
  Demux2/3 -> Bus Creator1/4  "Calf"
  Demux2/2 -> Bus Creator1/3  "Glut"
  Demux2/1 -> Bus Creator1/2  "Ham"
  Product1/1 -> Demux1/1
  Demux1/1 -> Bus Creator1/1  "Quad"
  Demux1/2 -> Bus Creator3/1  "Quad"

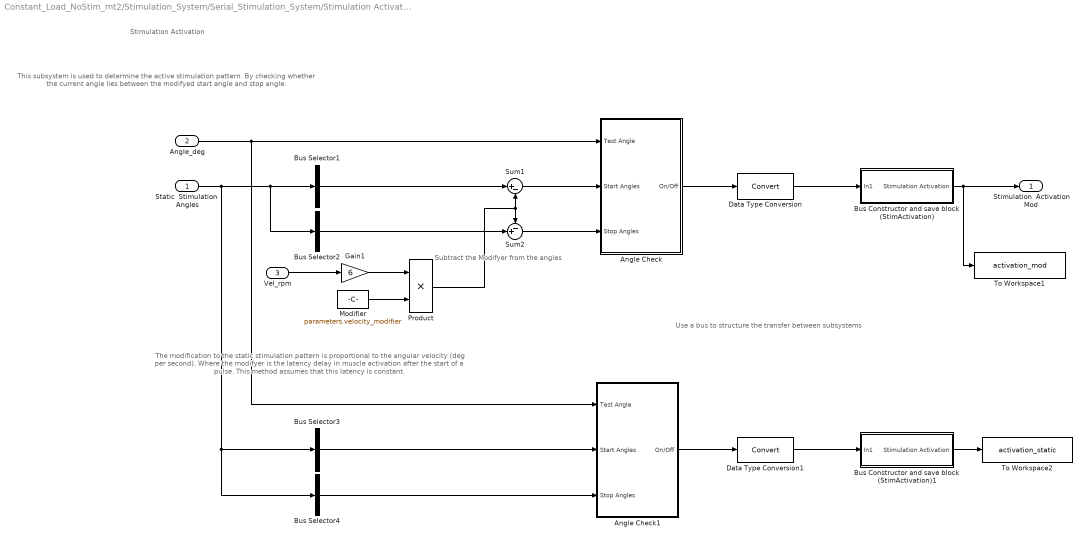
== system Constant_Load_NoStim_mt2/Stimulation_System/Serial_Stimulation_System/Stimulation Activation ==
  note: Stimulation Activation
  note: This subsystem is used to
      | determine the active stimulation
      | pattern.  By checking whether the
      | current angle lies between the modifyed
      | start angle and stop angle.
  note: Subtract the Modifyer
      | from the angles
  note: The modification to the static stimulation
      | pattern is proportional to the angular
      | velocity (deg per second).  Where the
      | modifyer is the latency delay in muscle
      | activation after the start of a pulse.  This
      | method assumes that this latency is
      | constant.
  note: Use a bus to structure the
      | transfer between subsystems
  Static  Stimulation  Angles : Inport
  Angle_deg : Inport  Port=2
  Vel_rpm : Inport  Port=3
  Angle Check : Subsystem
  Angle Check1 : Subsystem
  Bus Selector1 : BusSelector  OutputSignals=R.Quad.start,R.Ham.start,R.Glut.start,R.Calf.start,L.Quad.start,L.Ham.start,L.Glut.start,L.Calf.start  OutputAsBus=on
  Bus Selector2 : BusSelector  OutputSignals=R.Quad.stop,R.Ham.stop,R.Glut.stop,R.Calf.stop,L.Quad.stop,L.Ham.stop,L.Glut.stop,L.Calf.stop  OutputAsBus=on
  Bus Selector3 : BusSelector  OutputSignals=R.Quad.start,R.Ham.start,R.Glut.start,R.Calf.start,L.Quad.start,L.Ham.start,L.Glut.start,L.Calf.start  OutputAsBus=on
  Bus Selector4 : BusSelector  OutputSignals=R.Quad.stop,R.Ham.stop,R.Glut.stop,R.Calf.stop,L.Quad.stop,L.Ham.stop,L.Glut.stop,L.Calf.stop  OutputAsBus=on
  Bus Constructor and save block (StimActivation) : Subsystem
  Bus Constructor and save block (StimActivation)1 : Subsystem
  Data Type Conversion : DataTypeConversion  OutDataTypeMode=double
  Data Type Conversion1 : DataTypeConversion  OutDataTypeMode=double
  Gain1 : Gain  Gain=6  SaturateOnIntegerOverflow=on
  Modifier : Constant  Value=parameters.velocity_modifier
  Product : Product  SaturateOnIntegerOverflow=on  InputSameDT=on
  Sum1 : Sum  Inputs=|+-  SaturateOnIntegerOverflow=on  InputSameDT=on
  Sum2 : Sum  Inputs=-+|  SaturateOnIntegerOverflow=on  InputSameDT=on
  To Workspace1 : ToWorkspace  VariableName=activation_mod  SampleTime=parameters.model.sample_time  SaveFormat=Array
      settings: Decimation=5
  To Workspace2 : ToWorkspace  VariableName=activation_static  SampleTime=parameters.model.sample_time  SaveFormat=Array
      settings: Decimation=5
  Stimulation  Activation Mod : Outport
  wires:
  Angle_deg/1 -> Angle Check/1(Test Angle), Angle Check1/1(Test Angle)
  Static  Stimulation  Angles/1 -> Bus Selector1/1, Bus Selector2/1, Bus Selector3/1, Bus Selector4/1
  Vel_rpm/1 -> Gain1/1
  Modifier/1 -> Product/2
  Bus Constructor and save block (StimActivation)/1(Stimulation Activation) -> Stimulation  Activation Mod/1, To Workspace1/1
  Gain1/1 -> Product/1
  Data Type Conversion/1 -> Bus Constructor and save block (StimActivation)/1(In1)
  Angle Check/1(On/Off) -> Data Type Conversion/1
  Bus Selector1/1 -> Sum1/1
  Bus Selector2/1 -> Sum2/2
  Product/1 -> Sum2/1, Sum1/2
  Sum1/1 -> Angle Check/2(Start Angles)
  Sum2/1 -> Angle Check/3(Stop Angles)
  Bus Selector3/1 -> Angle Check1/2(Start Angles)
  Bus Selector4/1 -> Angle Check1/3(Stop Angles)
  Angle Check1/1(On/Off) -> Data Type Conversion1/1
  Data Type Conversion1/1 -> Bus Constructor and save block (StimActivation)1/1(In1)
  Bus Constructor and save block (StimActivation)1/1(Stimulation Activation) -> To Workspace2/1

== system Constant_Load_NoStim_mt2/Stimulation_System/Serial_Stimulation_System/Stimulator ==
  Current : Inport
  PW : Inport  Port=2
  Constant : Constant  Value=[0 0]
  Selector : Selector  IndexOptions=Index vector (dialog)  Indices=[1 4]  OutputSizes=1  InputPortWidth=6
  Selector1 : Selector  IndexOptions=Index vector (dialog)  Indices=[1 4]  OutputSizes=1  InputPortWidth=6
  Terminator1 : Terminator
  Terminator2 : Terminator
  Terminator3 : Terminator
  wires:
  Current/1 -> Selector1/1
  PW/1 -> Selector/1
  Selector1/1 -> Terminator3/1
  Selector/1 -> Terminator2/1
  Constant/1 -> Terminator1/1

== system Constant_Load_NoStim_mt2/Stimulation_System/Serial_Stimulation_System/Pulsewidth Generator/Intensity Modulation ==
  PW_ref : Inport
  Demux2 : Demux  Outputs=2
  Limit max PW : Saturate  UpperLimit=500  LowerLimit=0
  Limit max PW1 : Saturate  UpperLimit=500  LowerLimit=0
  To Workspace1 : ToWorkspace  VariableName=pulsewidth_ref_Q  SampleTime=parameters.model.sample_time  SaveFormat=Array
      settings: Decimation=5
  To Workspace2 : ToWorkspace  VariableName=pulsewidth_ref  SampleTime=parameters.model.sample_time  SaveFormat=Array
      settings: Decimation=5
  PW_Q : Outport
  PW : Outport  Port=2
  wires:
  PW_ref/1 -> Demux2/1  "PW_ref"
  Demux2/1 -> Limit max PW/1
  Demux2/2 -> Limit max PW1/1
  Limit max PW/1 -> PW_Q/1, To Workspace1/1  "Pulsewidth"
  Limit max PW1/1 -> PW/1, To Workspace2/1

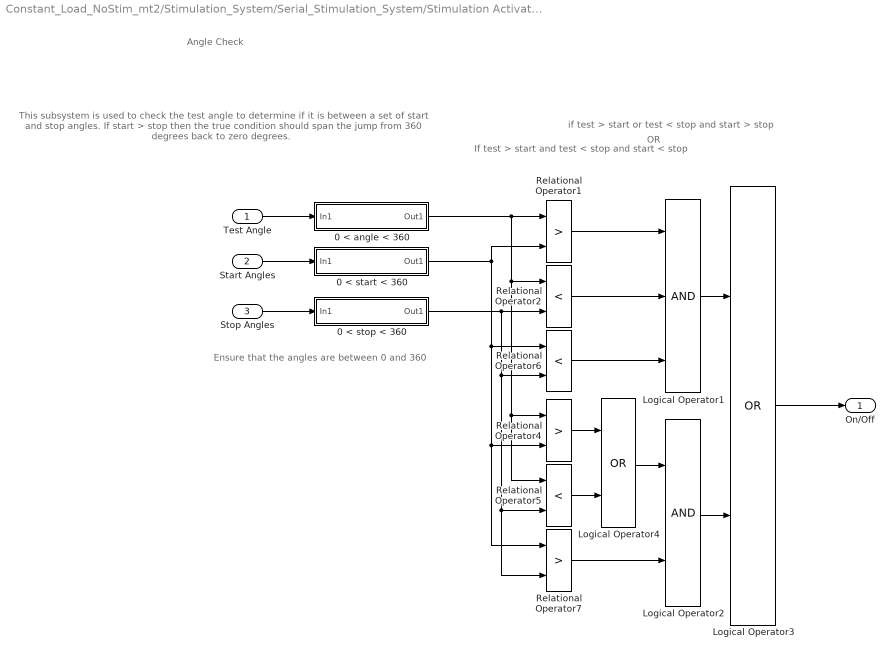
== system Constant_Load_NoStim_mt2/Stimulation_System/Serial_Stimulation_System/Stimulation Activation/Angle Check ==
  note: This subsystem is used to check
      | the test angle to determine if it is
      | between a set of  start and stop
      | angles.  If start > stop then the
      | true condition should span the
      | jump from 360 degrees back to
      | zero degrees.
  note: Angle Check
  note: OR
  note: if
      |   test > start
      |   or
      |   test < stop
      | and
      |   start > stop
  note: Ensure that the angles are
      | between 0 and 360
  note: If
      |   test > start
      | and
      |   test < stop
      | and
      |   start < stop
  Test Angle : Inport
  Start Angles : Inport  Port=2
  Stop Angles : Inport  Port=3
  0 < angle < 360 : Subsystem
  0 < start < 360 : Subsystem
  0 < stop < 360 : Subsystem
  Logical Operator1 : Logic  Inputs=3
  Logical Operator2 : Logic
  Logical Operator3 : Logic  Operator=OR
  Logical Operator4 : Logic  Operator=OR
  Relational Operator1 : RelationalOperator  Operator=>  InputSameDT=on
  Relational Operator2 : RelationalOperator  Operator=<  InputSameDT=on
  Relational Operator4 : RelationalOperator  Operator=>  InputSameDT=on
  Relational Operator5 : RelationalOperator  Operator=<  InputSameDT=on
  Relational Operator6 : RelationalOperator  Operator=<  InputSameDT=on
  Relational Operator7 : RelationalOperator  Operator=>  InputSameDT=on
  On/Off : Outport
  wires:
  Logical Operator4/1 -> Logical Operator2/1
  Relational Operator5/1 -> Logical Operator4/2
  Relational Operator4/1 -> Logical Operator4/1
  Logical Operator3/1 -> On/Off/1
  Logical Operator2/1 -> Logical Operator3/2
  Logical Operator1/1 -> Logical Operator3/1
  Relational Operator7/1 -> Logical Operator2/2
  Relational Operator6/1 -> Logical Operator1/3
  0 < stop < 360/1(Out1) -> Relational Operator2/2, Relational Operator7/2, Relational Operator5/2, Relational Operator6/2
  0 < angle < 360/1(Out1) -> Relational Operator2/1, Relational Operator5/1, Relational Operator4/1, Relational Operator1/1
  Stop Angles/1 -> 0 < stop < 360/1(In1)
  Start Angles/1 -> 0 < start < 360/1(In1)
  0 < start < 360/1(Out1) -> Relational Operator7/1, Relational Operator4/2, Relational Operator6/1, Relational Operator1/2
  Test Angle/1 -> 0 < angle < 360/1(In1)
  Relational Operator1/1 -> Logical Operator1/1
  Relational Operator2/1 -> Logical Operator1/2

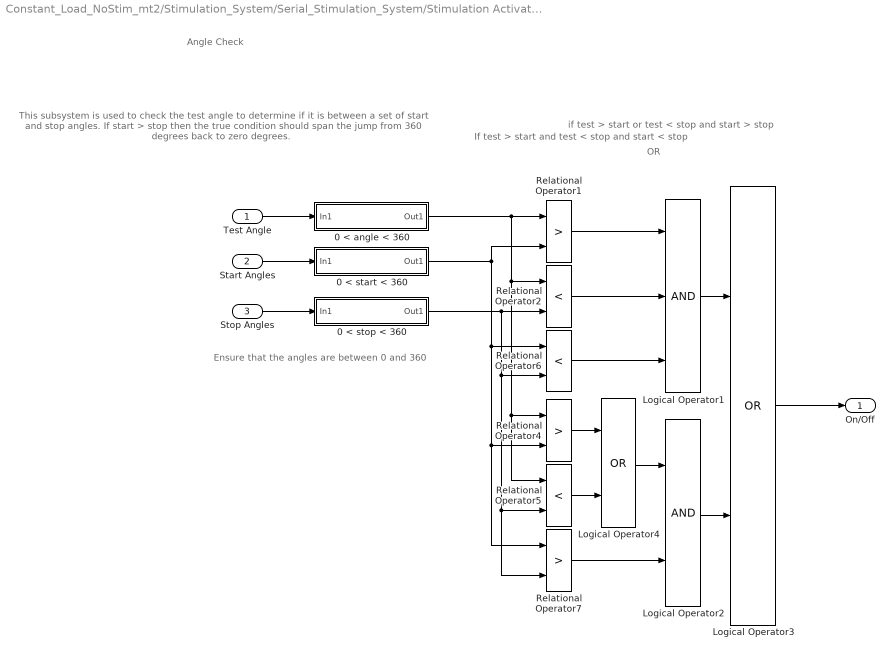
== system Constant_Load_NoStim_mt2/Stimulation_System/Serial_Stimulation_System/Stimulation Activation/Angle Check1 ==
  note: If
      |   test > start
      | and
      |   test < stop
      | and
      |   start < stop
  note: Ensure that the angles are
      | between 0 and 360
  note: if
      |   test > start
      |   or
      |   test < stop
      | and
      |   start > stop
  note: OR
  note: Angle Check
  note: This subsystem is used to check
      | the test angle to determine if it is
      | between a set of  start and stop
      | angles.  If start > stop then the
      | true condition should span the
      | jump from 360 degrees back to
      | zero degrees.
  Test Angle : Inport
  Start Angles : Inport  Port=2
  Stop Angles : Inport  Port=3
  0 < angle < 360 : Subsystem
  0 < start < 360 : Subsystem
  0 < stop < 360 : Subsystem
  Logical Operator1 : Logic  Inputs=3
  Logical Operator2 : Logic
  Logical Operator3 : Logic  Operator=OR
  Logical Operator4 : Logic  Operator=OR
  Relational Operator1 : RelationalOperator  Operator=>  InputSameDT=on
  Relational Operator2 : RelationalOperator  Operator=<  InputSameDT=on
  Relational Operator4 : RelationalOperator  Operator=>  InputSameDT=on
  Relational Operator5 : RelationalOperator  Operator=<  InputSameDT=on
  Relational Operator6 : RelationalOperator  Operator=<  InputSameDT=on
  Relational Operator7 : RelationalOperator  Operator=>  InputSameDT=on
  On/Off : Outport
  wires:
  Relational Operator2/1 -> Logical Operator1/2
  Relational Operator1/1 -> Logical Operator1/1
  Test Angle/1 -> 0 < angle < 360/1(In1)
  0 < start < 360/1(Out1) -> Relational Operator1/2, Relational Operator6/1, Relational Operator4/2, Relational Operator7/1
  Start Angles/1 -> 0 < start < 360/1(In1)
  Stop Angles/1 -> 0 < stop < 360/1(In1)
  0 < angle < 360/1(Out1) -> Relational Operator1/1, Relational Operator4/1, Relational Operator5/1, Relational Operator2/1
  0 < stop < 360/1(Out1) -> Relational Operator6/2, Relational Operator5/2, Relational Operator7/2, Relational Operator2/2
  Relational Operator6/1 -> Logical Operator1/3
  Relational Operator7/1 -> Logical Operator2/2
  Logical Operator1/1 -> Logical Operator3/1
  Logical Operator2/1 -> Logical Operator3/2
  Logical Operator3/1 -> On/Off/1
  Relational Operator4/1 -> Logical Operator4/1
  Relational Operator5/1 -> Logical Operator4/2
  Logical Operator4/1 -> Logical Operator2/1

== system Constant_Load_NoStim_mt2/Stimulation_System/Serial_Stimulation_System/Stimulation Activation/Bus Constructor and save block (StimActivation) ==
  note: Use a bus to structure the
      | transfer between subsystems
  note: Bus Constructor (StimActivation)
  In1 : Inport
  Bus Creator1 : BusCreator
  Bus Creator2 : BusCreator  Inputs=2
  Bus Creator3 : BusCreator
  Demux1 : Demux  Outputs=8
  Stimulation Activation : Outport
  wires:
  Demux1/8 -> Bus Creator3/4  "Calf"
  Demux1/7 -> Bus Creator3/3  "Glut"
  Demux1/6 -> Bus Creator3/2  "Ham"
  Demux1/5 -> Bus Creator3/1  "Quad"
  Demux1/4 -> Bus Creator1/4  "Calf"
  Demux1/3 -> Bus Creator1/3  "Glut"
  Demux1/2 -> Bus Creator1/2  "Ham"
  Demux1/1 -> Bus Creator1/1  "Quad"
  Bus Creator1/1 -> Bus Creator2/1  "R"
  Bus Creator3/1 -> Bus Creator2/2  "L"
  In1/1 -> Demux1/1
  Bus Creator2/1 -> Stimulation Activation/1  "Stimulation Activation"

== system Constant_Load_NoStim_mt2/Stimulation_System/Serial_Stimulation_System/Stimulation Activation/Bus Constructor and save block (StimActivation)1 ==
  note: Bus Constructor (StimActivation)
  note: Use a bus to structure the
      | transfer between subsystems
  In1 : Inport
  Bus Creator1 : BusCreator
  Bus Creator2 : BusCreator  Inputs=2
  Bus Creator3 : BusCreator
  Demux1 : Demux  Outputs=8
  Stimulation Activation : Outport
  wires:
  Bus Creator2/1 -> Stimulation Activation/1  "Stimulation Activation"
  In1/1 -> Demux1/1
  Bus Creator3/1 -> Bus Creator2/2  "L"
  Bus Creator1/1 -> Bus Creator2/1  "R"
  Demux1/1 -> Bus Creator1/1  "Quad"
  Demux1/2 -> Bus Creator1/2  "Ham"
  Demux1/3 -> Bus Creator1/3  "Glut"
  Demux1/4 -> Bus Creator1/4  "Calf"
  Demux1/5 -> Bus Creator3/1  "Quad"
  Demux1/6 -> Bus Creator3/2  "Ham"
  Demux1/7 -> Bus Creator3/3  "Glut"
  Demux1/8 -> Bus Creator3/4  "Calf"

== system Constant_Load_NoStim_mt2/Stimulation_System/Serial_Stimulation_System/Stimulation Activation/Angle Check/0 < angle < 360 ==
  In1 : Inport
  Gain : Gain  Gain=360  SaturateOnIntegerOverflow=on
  Gain1 : Gain  Gain=1/360  SaturateOnIntegerOverflow=on
  Rounding Function : Rounding
  Sum : Sum  Inputs=|+-  SaturateOnIntegerOverflow=on  InputSameDT=on
  Out1 : Outport
  wires:
  In1/1 -> Sum/1, Gain1/1
  Gain1/1 -> Rounding Function/1
  Rounding Function/1 -> Gain/1
  Gain/1 -> Sum/2
  Sum/1 -> Out1/1

== system Constant_Load_NoStim_mt2/Stimulation_System/Serial_Stimulation_System/Stimulation Activation/Angle Check/0 < start < 360 ==
  In1 : Inport
  Gain : Gain  Gain=360  SaturateOnIntegerOverflow=on
  Gain1 : Gain  Gain=1/360  SaturateOnIntegerOverflow=on
  Rounding Function : Rounding
  Sum : Sum  Inputs=|+-  SaturateOnIntegerOverflow=on  InputSameDT=on
  Out1 : Outport
  wires:
  Sum/1 -> Out1/1
  Gain/1 -> Sum/2
  Rounding Function/1 -> Gain/1
  Gain1/1 -> Rounding Function/1
  In1/1 -> Gain1/1, Sum/1

== system Constant_Load_NoStim_mt2/Stimulation_System/Serial_Stimulation_System/Stimulation Activation/Angle Check/0 < stop < 360 ==
  In1 : Inport
  Gain : Gain  Gain=360  SaturateOnIntegerOverflow=on
  Gain1 : Gain  Gain=1/360  SaturateOnIntegerOverflow=on
  Rounding Function : Rounding
  Sum : Sum  Inputs=|+-  SaturateOnIntegerOverflow=on  InputSameDT=on
  Out1 : Outport
  wires:
  In1/1 -> Sum/1, Gain1/1
  Gain1/1 -> Rounding Function/1
  Rounding Function/1 -> Gain/1
  Gain/1 -> Sum/2
  Sum/1 -> Out1/1

== system Constant_Load_NoStim_mt2/Stimulation_System/Serial_Stimulation_System/Stimulation Activation/Angle Check1/0 < angle < 360 ==
  In1 : Inport
  Gain : Gain  Gain=360  SaturateOnIntegerOverflow=on
  Gain1 : Gain  Gain=1/360  SaturateOnIntegerOverflow=on
  Rounding Function : Rounding
  Sum : Sum  Inputs=|+-  SaturateOnIntegerOverflow=on  InputSameDT=on
  Out1 : Outport
  wires:
  Sum/1 -> Out1/1
  Gain/1 -> Sum/2
  Rounding Function/1 -> Gain/1
  Gain1/1 -> Rounding Function/1
  In1/1 -> Gain1/1, Sum/1

== system Constant_Load_NoStim_mt2/Stimulation_System/Serial_Stimulation_System/Stimulation Activation/Angle Check1/0 < start < 360 ==
  In1 : Inport
  Gain : Gain  Gain=360  SaturateOnIntegerOverflow=on
  Gain1 : Gain  Gain=1/360  SaturateOnIntegerOverflow=on
  Rounding Function : Rounding
  Sum : Sum  Inputs=|+-  SaturateOnIntegerOverflow=on  InputSameDT=on
  Out1 : Outport
  wires:
  In1/1 -> Sum/1, Gain1/1
  Gain1/1 -> Rounding Function/1
  Rounding Function/1 -> Gain/1
  Gain/1 -> Sum/2
  Sum/1 -> Out1/1

== system Constant_Load_NoStim_mt2/Stimulation_System/Serial_Stimulation_System/Stimulation Activation/Angle Check1/0 < stop < 360 ==
  In1 : Inport
  Gain : Gain  Gain=360  SaturateOnIntegerOverflow=on
  Gain1 : Gain  Gain=1/360  SaturateOnIntegerOverflow=on
  Rounding Function : Rounding
  Sum : Sum  Inputs=|+-  SaturateOnIntegerOverflow=on  InputSameDT=on
  Out1 : Outport
  wires:
  Sum/1 -> Out1/1
  Gain/1 -> Sum/2
  Rounding Function/1 -> Gain/1
  Gain1/1 -> Rounding Function/1
  In1/1 -> Gain1/1, Sum/1
